simulink model "car_sim_for_student_r2015"  (R2022b)
settings: Solver=FixedStepAuto  StartTime=0.0  StopTime=40  FixedStep=0.001  RelTol=1e-3
InitFcn:
  | load('sysu_standard.mat');
  | load('traj_diySYSU.mat');
values from neighbouring files (symbols this model uses):
  map = ~inflatedMap    [temp.m]
  trajSYSU = path    [temp.m]
undefined symbols (not defined in the file or in its folder): gray, out
libraries: slpidlib x1, simulink x1
settings Model: Creator=Manny  LastModifiedBy=秦华谦
settings SolverCC: AlgebraicLoopSolver=LineSearch
settings OptimizationCC: LifeSpan=inf
settings DebuggingCC: UnconnectedInputMsg=warning  UnconnectedOutputMsg=warning  UnconnectedLineMsg=warning  SFExecutionAtInitializationDiag=none  SFMachineParentedDataDiag=warning  ArithmeticOperatorsInVariantConditions=warning
settings ModelReferenceCC: EnableRefExpFcnMdlSchedulingChecks=on
settings SFSimCC: CustomCodeUndefinedFunction=UseInterfaceOnly
settings CodeAppCC: StateflowObjectComments=on

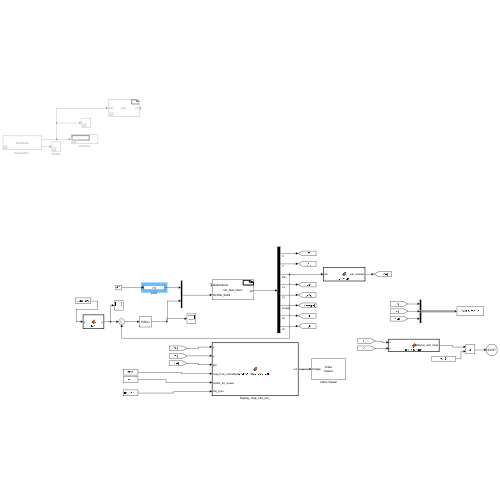
[thumbnail: Simulink's stored preview of the top-level diagram]
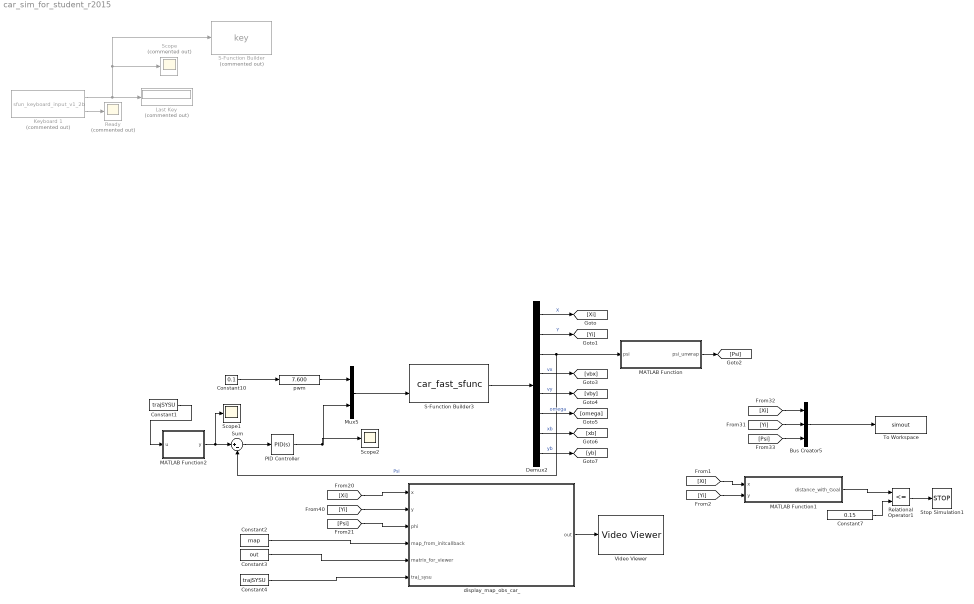
== system car_sim_for_student_r2015 ==
  Bus Creator5 : BusCreator  Inputs=3
  Constant1 : Constant  Value=trajSYSU
  Constant10 : Constant  Value=0.1
  Constant2 : Constant  Value=map
  Constant3 : Constant  Value=out
  Constant4 : Constant  Value=trajSYSU
  Constant7 : Constant  Value=0.15
  Demux2 : Demux  Outputs=8
  Keyboard 1 : M-S-Function  Commented=on  FunctionName=sfun_keyboard_input_v1_2b  mask(Keyboard Input){}
      mask help: Keyboard Input
      mask Display: fprintf('Keyboard');
  Last Key : Display  Commented=on
  MATLAB Function : MATLAB Function  TreatAsAtomicUnit=on
  MATLAB Function1 : MATLAB Function  TreatAsAtomicUnit=on
  MATLAB Function2 : MATLAB Function  TreatAsAtomicUnit=on
  Mux5 : Mux  Inputs=2
  PID Controller : slpidlib/PID Controller  Controller=PID  Form=Parallel  TimeDomain=Continuous-time  UseExternalTs=off  SampleTime=-1  IntegratorMethod=Forward Euler  FilterMethod=Forward Euler  ControllerParametersSource=internal  P=5  I=1  UseKiTs=off  D=0.1  N=100  UseFilter=on  TunerSelectOption=Transfer Function Based (PID Tuner App)  InitialConditionSource=internal  InitialConditionForIntegrator=0  InitialConditionForFilter=0  DifferentiatorICPrevScaledInput=0  ExternalReset=none  TrackingMode=off  Kt=1  LimitOutput=off  SatLimitsSource=internal  UpperSaturationLimit=inf  LowerSaturationLimit=-inf  LinearizeAsGain=on  AntiWindupMode=none  Kb=1  LimitIntegrator=off  UpperIntegratorSaturationLimit=inf  LowerIntegratorSaturationLimit=-inf  POutMin=[]  POutMax=[]  IOutMin=[]  IOutMax=[]  DOutMin=[]  DOutMax=[]  NOutMin=[]  NOutMax=[]  SumOutMin=[]  SumOutMax=[]  SaturationOutMin=[]  SaturationOutMax=[]  PParamMin=[]  PParamMax=[]  IParamMin=[]  IParamMax=[]  DParamMin=[]  DParamMax=[]  NParamMin=[]  NParamMax=[]  KbParamMin=[]  KbParamMax=[]  KtParamMin=[]  KtParamMax=[]  KbOutMin=[]  KbOutMax=[]  KtOutMin=[]  KtOutMax=[]  IntegratorOutMin=[]  IntegratorOutMax=[]  FilterOutMin=[]  FilterOutMax=[]  SumI1OutMin=[]  SumI1OutMax=[]  SumI2OutMin=[]  SumI2OutMax=[]  SumI3OutMin=[]  SumI3OutMax=[]  SumI4OutMin=[]  SumI4OutMax=[]  SumDOutMin=[]  SumDOutMax=[]  DifferentiatorOutMin=[]  DifferentiatorOutMax=[]  FilterDiffOutCoefMin=[]  FilterDiffOutCoefMax=[]  ReciprocalOutMin=[]  ReciprocalOutMax=[]  SumDenOutMin=[]  SumDenOutMax=[]  SumNumOutMin=[]  SumNumOutMax=[]  DivideOutMin=[]  DivideOutMax=[]  UdiffTsProdOutMin=[]  UdiffTsProdOutMax=[]  NTsProdOutMin=[]  NTsProdOutMax=[]  UintegralTsProdOutMin=[]  UintegralTsProdOutMax=[]  UngainTsProdOutMin=[]  UngainTsProdOutMax=[]  ClampingZeroOutDataTypeStr=Inherit: Inherit via back propagation  ClampingZeroOutMin=[]  ClampingZeroOutMax=[]  FilterDenConstantOutDataTypeStr=Inherit: Inherit via back propagation  FilterDenConstantOutMin=[]  FilterDenConstantOutMax=[]  PCopyOutDataTypeStr=Inherit: Inherit via back propagation  PCopyOutMin=[]  PCopyOutMax=[]  NCopyOutDataTypeStr=Inherit: Inherit via back propagation  NCopyOutMin=[]  NCopyOutMax=[]  IntegratorContinuousStateAttributes=''  IntegratorStateMustResolveToSignalObject=off  IntegratorRTWStateStorageClass=Auto  FilterContinuousStateAttributes=''  FilterStateMustResolveToSignalObject=off  FilterRTWStateStorageClass=Auto  ParallelPVariant=InternalParameters  IdealPVariant=Disabled  IVariant=InternalParameters  DVariant=InternalParameters  IntegratorVariant=Continuous  SatVariant=Disabled  AWVariant=Passthrough  PCopyVariant=Disabled  TRVariant=Disabled  FdbkBlocksVariant=Forward  IdealPFdbkVariant=Disabled  SatFdbkVariant=Disabled  DerivativeFilterVariant=ContFilter  NVariant=InternalParameters  NCopyVariant=Disabled  FilterICVariant=InternalICsFilter  IntegratorICVariant=InternalICs  ExternalResetVariant=Disabled  TRSumVariant=Passthrough  SumFdbkVariant=Disabled  SumVariant=Sum_PID  TsampFilterVariant=InternalTs  TsampNgainVariant=Passthrough  TsampIntegralVariant=Passthrough  ExternalSaturationOutDataTypeStr=Inherit: Same as second input
  Ready : Scope  Commented=on
  Relational Operator1 : RelationalOperator  Operator=<=  OutDataTypeStr=boolean  InputSameDT=off
  S-Function Builder : S-Function  Commented=on  FunctionName=key  SFunctionModules=key_wrapper  SFunctionDeploymentMode=off  EnableBusSupport=off  mask(S-Function Builder){}
      mask help: Simulink:masks:SFunctionBuilder_MD
      mask init:
      | val = [[.9  0.75 0.75 1 1 .9 .9 1]',[1 1 0.75 0.75 .9 .9 1 .9]'];try , sys = get_param(gcb,'SfunBuilderFcnName');if isempty(sys), sys = get_param(gcb,'FunctionName'); end,catch, sys = get_param(gcb,'FunctionName'); end
      settings: CopyFcn=set_param(gcbh,'LinkStatus','none')  OpenFcn=sfunctionwizard(gcbh)
      mask Display:
      | plot(val(:,1),val(:,2))
      | disp(sys)
      | port_label('input',1,'key')
      | port_label('output',1,'y0')
  S-Function Builder3 : S-Function  FunctionName=car_fast_sfunc  SFunctionModules=car_fast_sfunc_wrapper  SFunctionDeploymentMode=off  EnableBusSupport=off  mask(S-Function Builder){}
      mask help: Simulink:masks:SFunctionBuilder_MD
      mask init: same as car_sim_for_student_r2015/S-Function Builder
      settings: CopyFcn=set_param(gcbh,'LinkStatus','none')  OpenFcn=sfunctionwizard(gcbh)
      mask Display:
      | plot(val(:,1),val(:,2))
      | disp(sys)
      | port_label('input',1,'disturbance')
      | port_label('input',2,'throttle_delta')
      | port_label('output',1,'y0')
  Scope : Scope  Commented=on
  Scope1 : Scope
  Scope2 : Scope
  Stop Simulation1 : Stop
  Sum : Sum  Inputs=|+-
  To Workspace : ToWorkspace  VariableName=simout  SaveFormat=Timeseries  SampleTime=-1
  Video Viewer : VideoViewer  colormapValue=gray(256)  FigPos=[278.6 736.4 1055.2 498.4]
  display_map_obs_car_ : MATLAB Function  TreatAsAtomicUnit=on
  pwm : simulink/Math Operations/Slider Gain  gain=7.600  low=-20  high=20
  wires:
  S-Function Builder3/1 -> Demux2/1
  Demux2/2 -> [Yi]  "Y"
  Demux2/3 -> Sum/2, MATLAB Function/1(psi)  "Psi"
  Demux2/4 -> [vbx]  "vx"
  Demux2/5 -> [vby]  "vy"
  Demux2/6 -> [omega]  "omega"
  Demux2/7 -> [xb]  "xb"
  Demux2/8 -> [yb]  "yb"
  MATLAB Function/1(psi_unwrap) -> [Psi]
  [Yi] -> display_map_obs_car_/2(y)
  [Xi] -> display_map_obs_car_/1(x)
  [Psi] -> display_map_obs_car_/3(phi)
  display_map_obs_car_/1(out) -> Video Viewer/1
  Constant2/1 -> display_map_obs_car_/4(map_from_initcallback)
  Demux2/1 -> [Xi]  "X"
  Constant3/1 -> display_map_obs_car_/5(matrix_for_viewer)
  Constant10/1 -> pwm/1
  pwm/1 -> Mux5/1
  Keyboard 1/1 -> S-Function Builder/1, Scope/1, Last Key/1
  Keyboard 1/2 -> Ready/1
  [Yi] -> Bus Creator5/2
  Bus Creator5/1 -> To Workspace/1
  [Psi] -> Bus Creator5/3
  [Xi] -> Bus Creator5/1
  Constant4/1 -> display_map_obs_car_/6(traj_sysu)
  Mux5/1 -> S-Function Builder3/2
  [Xi] -> MATLAB Function1/1(x)
  MATLAB Function1/1(distance_with_Goal) -> Relational Operator1/1
  Relational Operator1/1 -> Stop Simulation1/1
  Constant7/1 -> Relational Operator1/2
  [Yi] -> MATLAB Function1/2(y)
  Constant1/1 -> MATLAB Function2/1(u)
  MATLAB Function2/1(y) -> Scope1/1, Sum/1
  Sum/1 -> PID Controller/1
  PID Controller/1 -> Scope2/1, Mux5/2

== matlab function car_sim_for_student_r2015/MATLAB Function1 ==
  data: x input; distance_with_Goal output; y input
function distance_with_Goal = cal_distance(x,y)
distance_with_Goal=sqrt((x-11.3)*(x-11.3)+(y-4.5)*(y-4.5))

== matlab function car_sim_for_student_r2015/display_map_obs_car_ ==
  settings: updateMethod=DISCRETE
  data: x input; y input; phi input; out output size=600,1200,3; map_from_initcallback input size=600,1200; matrix_for_viewer input; traj_sysu input
function out = display_map_obs_car_(x,y,phi,map_from_initcallback,matrix_for_viewer,traj_sysu)
    persistent data;
    persistent times;
    if isempty(data)
        times=1;
    else
        times=times+1;
    end
    
    % 地图长12m 宽6m   车长0.12 车宽0.06
    resolution = 0.01;
    map_long=12;
    map_wide=6;

    car_long=0.12;
    car_wide=0.06;

    % 可视化地图
%     figure;
%     imagesc(map);%imagesc 可以将矩阵或数组的值映射到颜色图像中
%     colormap(flipud(gray));%colormap 将数据值映射到颜色空间中 colormap(flipud(gray)) 来设置颜色映射表为灰度图像。
    map=map_from_initcallback;    
    out=matrix_for_viewer;
    number_path=size(traj_sysu,2);
    for tmp=1:number_path
        traj_sysu_index=real2map([traj_sysu(1,tmp),traj_sysu(2,tmp)],map_wide,resolution);
        out(round(traj_sysu_index(1)+1/2),round(traj_sysu_index(2)+1/2),:)=[0,0,0];
    end
    x_now=x;%m  real视野坐标系,横着往右
    y_now=y;%m  real视野坐标系,竖着往上
    map_coord=real2map([x_now,y_now],map_wide,resolution);
    if isempty(data)
        data = zeros(99999, 2);
    else
        data(round(times/10)+1,:) = [map_coord(1),map_coord(2)];
        for times_disp_tmp=1:round(times/10)
            tmp_Data=data(times_disp_tmp,:);
            tmp_Data_next=data(times_disp_tmp+1,:);
%             out(round(tmp_Data(1,1)+1/2),round(tmp_Data(1,2)+1/2),:)=[0,0,1];

    
            vector=tmp_Data_next-tmp_Data;
            for t=0:0.025:1
                    new_point=tmp_Data+t*vector;
                    out(round(new_point(1)+1/2),round(new_point(2)+1/2),:)=[0,0,1];
                    out(round(new_point(1)+1/2),round(new_point(2)+1/2)-1,:)=[0,0,1];
                    out(round(new_point(1)+1/2),round(new_point(2)+1/2)+1,:)=[0,0,1];
            end

        end
    end



   
%     occ_or_not=get_occ_or_not(map_coord,map,resolution)
    occ_or_not=get_occ_or_not_Real([x_now,y_now],map_wide,map,resolution);
    l = car_long / resolution;
    w = car_wide / resolution;
    phi = phi; 




out=display_car(map_coord,phi,l,w,map,out);

%     axis equal;
%     axis off;
end

function occ_or_not=get_occ_or_not_Real(x_y,map_wide,map,resolution)
%round四舍五入 
map_coord=real2map(x_y,map_wide,resolution);
if(round(map_coord(1)+1/2)<1) ||(round(map_coord(1)+1/2)>600) ||(round(map_coord(2)+1/2)<1) ||(round(map_coord(2)+1/2)>1200)
    x_y
    disp('out of map');
end
 occ_or_not=map(round(map_coord(1)+1/2),round(map_coord(2)+1/2));
end
function occ_or_not=get_occ_or_not_map(map_coord,map,resolution)
%round四舍五入 
if(round(map_coord(1)+1/2)<1) ||(round(map_coord(1)+1/2)>600) ||(round(map_coord(2)+1/2)<1) ||(round(map_coord(2)+1/2)>1200)
    disp('out of map');
end
 occ_or_not=map(round(map_coord(1)+1/2),round(map_coord(2)+1/2));
end
function map_coord=real2map(x_y,map_wide,resolution)
    %地图向下是正x 向右是正y，
    % 因此在map上显示赛道小车障碍物的时候map_y直接取real世界的x, map_x需要把real_y反向并弄个静差
    map_coord=zeros(1,2);
    map_coord(1)=map_wide/ resolution-x_y(2)/ resolution;
    map_coord(2)=x_y(1)/ resolution ;
end

function matrix_for_viewer_new=display_car(map_coord,phi,l,w,map,matrix_for_viewer)
    %display是向右是x正，向下是y正
    pts = [
        map_coord(1)- [sin(phi)*l-cos(phi)*w, sin(phi)*l+cos(phi)*w,-sin(phi)*l+cos(phi)*w,-sin(phi)*l-cos(phi)*w]
        map_coord(2) + [cos(phi)*l+sin(phi)*w, cos(phi)*l-sin(phi)*w,-cos(phi)*l-sin(phi)*w,-cos(phi)*l+sin(phi)*w]
        
    ];
    map_index1=[round(pts(1,1)+1/2),round(pts(2,1)+1/2)];
    map_index2=[round(pts(1,2)+1/2),round(pts(2,2)+1/2)];
    map_index3=[round(pts(1,3)+1/2),round(pts(2,3)+1/2)];
    map_index4=[round(pts(1,4)+1/2),round(pts(2,4)+1/2)];

    matrix_for_viewer_new=matrix_for_viewer;
    %凸包，边缘线无碰撞则整体无碰撞
    have_somewhere_occ=0;
    vector_A_B=[map_index2(1)-map_index1(1),map_index2(2)-map_index1(2)];
    vector_A_D=[map_index4(1)-map_index1(1),map_index4(2)-map_index1(2)];
    for t1=0:0.025:1
        for t2=0:0.025:1
            new_point=map_index1+t1*vector_A_B+t2*vector_A_D;
            matrix_for_viewer_new(round(new_point(1)+0.5),round(new_point(2)+0.5),:)=[1,0,0];
            occ_or_not=map(round(new_point(1)+0.5),round(new_point(2)+0.5));
            if(occ_or_not==1)
               have_somewhere_occ=1;
           end
        end
    end
    if(have_somewhere_occ==1)
%         disp("collision!!");
    end
end

== matlab function car_sim_for_student_r2015/MATLAB Function ==
  data: psi input; psi_unwrap output
function psi_unwrap = unwrap(psi)

if ( psi > pi)
    psi = psi - 2*pi;
end

if( psi <= -pi)
    psi = psi + 2*pi;
end

psi_unwrap = psi;

== matlab function car_sim_for_student_r2015/MATLAB Function2 ==
  data: u input; y output
function y = fcn(u)

y = u(1);
